simulink model "model"  (R2015a)
settings: Solver=ode45  StartTime=0.0  StopTime=100  MaxStep=0.01  RelTol=1e-3
values from neighbouring files (symbols this model uses):
  e = 0.01    [Dyskretne.m]
  k = 7.95    [Dyskretne.m]
settings Model: Creator=pingwin  LastModifiedBy=pingwin

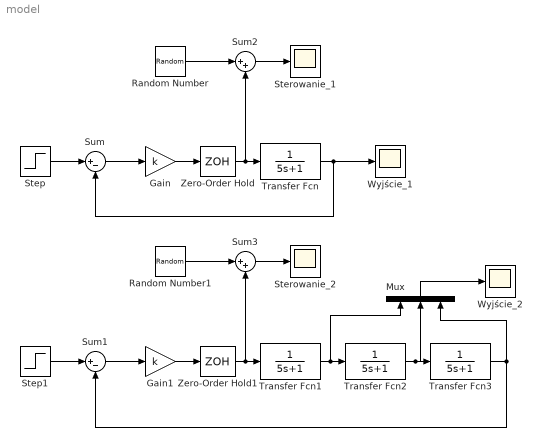
== system model ==
  Gain : Gain  Gain=k
  Gain1 : Gain  Gain=k
  Mux : Mux  Inputs=3
  Random Number : RandomNumber  Variance=0.0000001  SampleTime=0.01
  Random Number1 : RandomNumber  Variance=0.0000001  SampleTime=0.01
  Step : Step  SampleTime=0
  Step1 : Step  SampleTime=0
  Sterowanie_1 : Scope
      settings: SaveName=sterowanie_1  MaxDataPoints=5000000  SampleInput=on
  Sterowanie_2 : Scope
      settings: TimeRange=100  YMin=-2  SaveName=sterowanie_2  SampleInput=on
  Sum : Sum  Inputs=|+-
  Sum1 : Sum  Inputs=|+-
  Sum2 : Sum  Inputs=|++
  Sum3 : Sum  Inputs=|++
  Transfer Fcn{,1..3} (4 alike) : TransferFcn  Denominator=[5 1]
  Wyjście_1 : Scope
      settings: SaveName=output_1  MaxDataPoints=5000000  SampleInput=on
  Wyjście_2 : Scope
      settings: SaveName=output_2  SampleInput=on
  Zero-Order Hold : ZeroOrderHold  SampleTime=e
  Zero-Order Hold1 : ZeroOrderHold  SampleTime=e
  wires:
  Step/1 -> Sum/1
  Sum/1 -> Gain/1
  Gain/1 -> Zero-Order Hold/1
  Zero-Order Hold/1 -> Sum2/2, Transfer Fcn/1
  Step1/1 -> Sum1/1
  Sum1/1 -> Gain1/1
  Gain1/1 -> Zero-Order Hold1/1
  Zero-Order Hold1/1 -> Sum3/2, Transfer Fcn1/1
  Transfer Fcn1/1 -> Mux/1, Transfer Fcn2/1
  Transfer Fcn/1 -> Wyjście_1/1, Sum/2
  Transfer Fcn3/1 -> Mux/3, Sum1/2
  Transfer Fcn2/1 -> Mux/2, Transfer Fcn3/1
  Mux/1 -> Wyjście_2/1
  Random Number/1 -> Sum2/1
  Sum2/1 -> Sterowanie_1/1
  Random Number1/1 -> Sum3/1
  Sum3/1 -> Sterowanie_2/1
